simulink model "Ny_Model"  (R2016a)
settings: Solver=VariableStepAuto  StartTime=0.0  StopTime=3.5  RelTol=1e-3
values from neighbouring files (symbols this model uses):
  K = 651/12    (= 54.25)    [Model.m]    (also in PID_test.m = 96.2958333333; Rlocus.m = 0.0274)
  T = 0.014    [Model.m]    (also in PID_test.m = 0.12)
undefined symbols (not defined in the file or in its folder): k
libraries: simulink x2
settings Model: Creator=Kristian  LastModifiedBy=Kristian

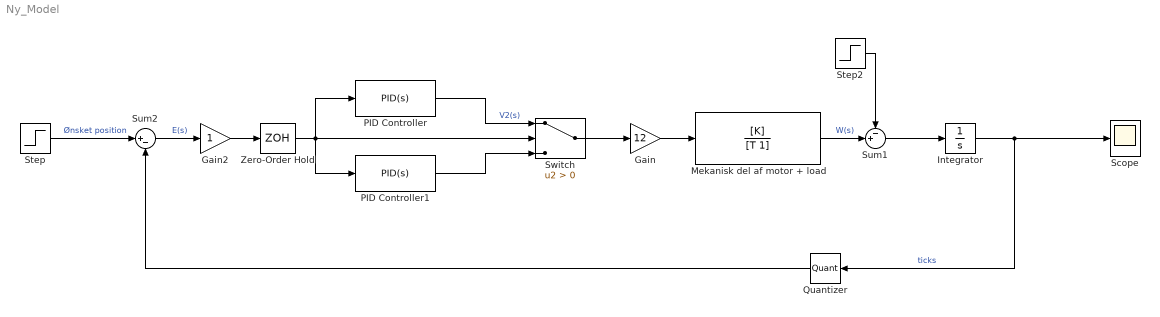
== system Ny_Model ==
  Gain : Gain  Gain=12
  Gain2 : Gain
  Integrator : Integrator
  "Mekanisk del af motor + load " : TransferFcn  Numerator=[K]  Denominator=[T 1]
  PID Controller : simulink/Continuous/PID Controller  Controller=PID  TimeDomain=Continuous-time  SampleTime=-1  IntegratorMethod=Forward Euler  FilterMethod=Forward Euler  Form=Parallel  UseFilter=off  ControllerParametersSource=internal  P=2*k  I=1*k  D=1*k  N=20  InitialConditionSource=internal  InitialConditionForIntegrator=0  InitialConditionForFilter=0  ExternalReset=none  IgnoreLimit=on  LimitOutput=on  UpperSaturationLimit=0.39  LowerSaturationLimit=0.16  LinearizeAsGain=on  AntiWindupMode=clamping  Kb=1  TrackingMode=off  Kt=1  SaturateOnIntegerOverflow=on  PParamMin=[]  PParamMax=[]  IParamMin=[]  IParamMax=[]  DParamMin=[]  DParamMax=[]  NParamMin=[]  NParamMax=[]  KbParamMin=[]  KbParamMax=[]  KtParamMin=[]  KtParamMax=[]  POutMin=[]  POutMax=[]  IOutMin=[]  IOutMax=[]  DOutMin=[]  DOutMax=[]  NOutMin=[]  NOutMax=[]  KbOutMin=[]  KbOutMax=[]  KtOutMin=[]  KtOutMax=[]  IntegratorOutMin=[]  IntegratorOutMax=[]  FilterOutMin=[]  FilterOutMax=[]  SumOutMin=[]  SumOutMax=[]  SumI1OutMin=[]  SumI1OutMax=[]  SumI2OutMin=[]  SumI2OutMax=[]  SumI3OutMin=[]  SumI3OutMax=[]  SumDOutMin=[]  SumDOutMax=[]  SaturationOutMin=[]  SaturationOutMax=[]  IntegratorContinuousStateAttributes=''  IntegratorStateMustResolveToSignalObject=off  IntegratorRTWStateStorageClass=Auto  FilterContinuousStateAttributes=''  FilterStateMustResolveToSignalObject=off  FilterRTWStateStorageClass=Auto  DifferentiatorICPrevScaledInput=0  DifferentiatorOutMin=[]  DifferentiatorOutMax=[]
  PID Controller1 : simulink/Continuous/PID Controller  Controller=PID  TimeDomain=Continuous-time  SampleTime=-1  IntegratorMethod=Forward Euler  FilterMethod=Forward Euler  Form=Parallel  UseFilter=off  ControllerParametersSource=internal  P=2*k  I=1*k  D=1*k  N=20  InitialConditionSource=internal  InitialConditionForIntegrator=0  InitialConditionForFilter=0  ExternalReset=none  IgnoreLimit=on  LimitOutput=on  UpperSaturationLimit=-0.16  LowerSaturationLimit=-0.39  LinearizeAsGain=on  AntiWindupMode=clamping  Kb=1  TrackingMode=off  Kt=1  SaturateOnIntegerOverflow=on  PParamMin=[]  PParamMax=[]  IParamMin=[]  IParamMax=[]  DParamMin=[]  DParamMax=[]  NParamMin=[]  NParamMax=[]  KbParamMin=[]  KbParamMax=[]  KtParamMin=[]  KtParamMax=[]  POutMin=[]  POutMax=[]  IOutMin=[]  IOutMax=[]  DOutMin=[]  DOutMax=[]  NOutMin=[]  NOutMax=[]  KbOutMin=[]  KbOutMax=[]  KtOutMin=[]  KtOutMax=[]  IntegratorOutMin=[]  IntegratorOutMax=[]  FilterOutMin=[]  FilterOutMax=[]  SumOutMin=[]  SumOutMax=[]  SumI1OutMin=[]  SumI1OutMax=[]  SumI2OutMin=[]  SumI2OutMax=[]  SumI3OutMin=[]  SumI3OutMax=[]  SumDOutMin=[]  SumDOutMax=[]  SaturationOutMin=[]  SaturationOutMax=[]  IntegratorContinuousStateAttributes=''  IntegratorStateMustResolveToSignalObject=off  IntegratorRTWStateStorageClass=Auto  FilterContinuousStateAttributes=''  FilterStateMustResolveToSignalObject=off  FilterRTWStateStorageClass=Auto  DifferentiatorICPrevScaledInput=0  DifferentiatorOutMin=[]  DifferentiatorOutMax=[]
  Quantizer : Quantizer  QuantizationInterval=1
  Scope : Scope
  "Step " : Step  Time=0  After=540  SampleTime=0
  Step2 : Step  Time=5  After=0  SampleTime=0
  Sum1 : Sum  Inputs=-+|
  Sum2 : Sum  Inputs=|+-
  Switch : Switch  Criteria=u2 > Threshold
  Zero-Order Hold : ZeroOrderHold  SampleTime=0.005
  wires:
  "Step "/1 -> Sum2/1  "Ønsket position"
  Gain/1 -> "Mekanisk del af motor + load "/1
  Sum2/1 -> Gain2/1  "E(s)"
  "Mekanisk del af motor + load "/1 -> Sum1/2  "W(s)"
  Sum1/1 -> Integrator/1
  Step2/1 -> Sum1/1
  Integrator/1 -> Scope/1, Quantizer/1  "ticks"
  Gain2/1 -> Zero-Order Hold/1
  PID Controller/1 -> Switch/1  "V2(s)"
  PID Controller1/1 -> Switch/3
  Switch/1 -> Gain/1
  Zero-Order Hold/1 -> PID Controller1/1, Switch/2, PID Controller/1
  Quantizer/1 -> Sum2/2
